simulink library "INT_PTODi_SpdCoord"  (R2016b)
settings: Solver=VariableStepAuto  StartTime=0.0  StopTime=10.0  RelTol=1e-3
settings Model: Creator=Administrator  LastModifiedBy=Administrator

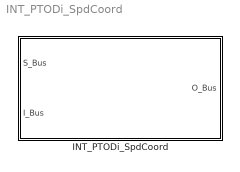
== system INT_PTODi_SpdCoord ==
  INT_PTODi_SpdCoord : Subsystem

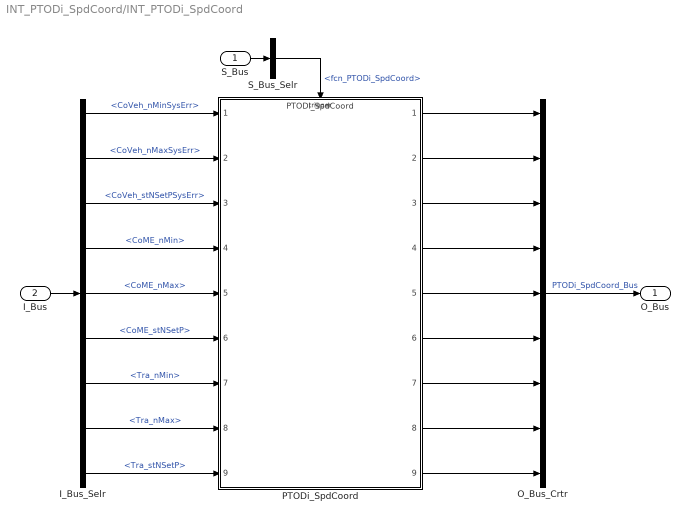
== system INT_PTODi_SpdCoord/INT_PTODi_SpdCoord ==
  S_Bus : Inport
  I_Bus : Inport  Port=2
  I_Bus_Selr : BusSelector  OutputSignals=CoVeh_nMinSysErr,CoVeh_nMaxSysErr,CoVeh_stNSetPSysErr,CoME_nMin,CoME_nMax,CoME_stNSetP,Tra_nMin,Tra_nMax,Tra_stNSetP
  O_Bus_Crtr : BusCreator  Inputs=9
  PTODi_SpdCoord : ModelReference  ModelNameDialog=PTODi_SpdCoord  SimulationMode=Normal  ModelReferenceVersion=1.3  TriggerPortName=function  TriggerPortTriggerType=function-call  TriggerPortStatesWhenEnabling=held
  S_Bus_Selr : BusSelector  OutputSignals=fcn_PTODi_SpdCoord
  O_Bus : Outport
  wires:
  S_Bus_Selr/1 -> PTODi_SpdCoord/Trigger  "<fcn_PTODi_SpdCoord>"
  S_Bus/1 -> S_Bus_Selr/1
  I_Bus/1 -> I_Bus_Selr/1
  I_Bus_Selr/1 -> PTODi_SpdCoord/1  "<CoVeh_nMinSysErr>"
  I_Bus_Selr/2 -> PTODi_SpdCoord/2  "<CoVeh_nMaxSysErr>"
  I_Bus_Selr/3 -> PTODi_SpdCoord/3  "<CoVeh_stNSetPSysErr>"
  I_Bus_Selr/4 -> PTODi_SpdCoord/4  "<CoME_nMin>"
  I_Bus_Selr/5 -> PTODi_SpdCoord/5  "<CoME_nMax>"
  I_Bus_Selr/6 -> PTODi_SpdCoord/6  "<CoME_stNSetP>"
  I_Bus_Selr/7 -> PTODi_SpdCoord/7  "<Tra_nMin>"
  I_Bus_Selr/8 -> PTODi_SpdCoord/8  "<Tra_nMax>"
  I_Bus_Selr/9 -> PTODi_SpdCoord/9  "<Tra_stNSetP>"
  O_Bus_Crtr/1 -> O_Bus/1  "PTODi_SpdCoord_Bus"
  PTODi_SpdCoord/1 -> O_Bus_Crtr/1
  PTODi_SpdCoord/2 -> O_Bus_Crtr/2
  PTODi_SpdCoord/3 -> O_Bus_Crtr/3
  PTODi_SpdCoord/4 -> O_Bus_Crtr/4
  PTODi_SpdCoord/5 -> O_Bus_Crtr/5
  PTODi_SpdCoord/6 -> O_Bus_Crtr/6
  PTODi_SpdCoord/7 -> O_Bus_Crtr/7
  PTODi_SpdCoord/8 -> O_Bus_Crtr/8
  PTODi_SpdCoord/9 -> O_Bus_Crtr/9
